simulink model "main_model"  (R2021b)
settings: Solver=ode4  StartTime=0.0  StopTime=7.0  FixedStep=rmpcProps.time_step  RelTol=1e-3
undefined symbols (not defined in the file): driverProps, refTraj, rmpcProps, vehProps
settings Model: Creator=vpurohi  LastModifiedBy=vpurohi

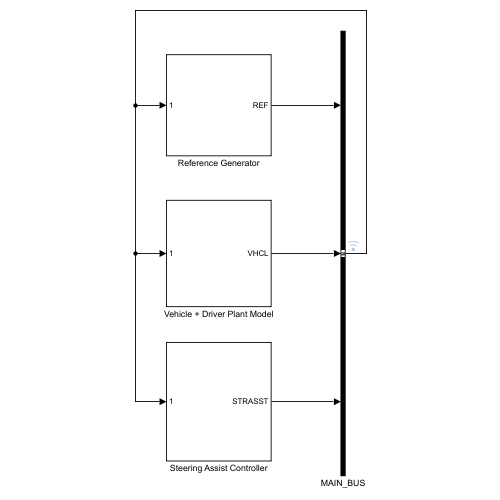
[thumbnail: Simulink's stored preview of the top-level diagram]
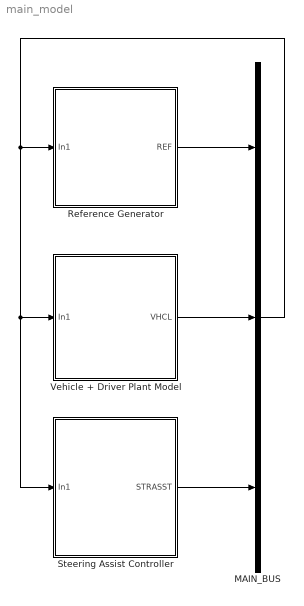
== system main_model ==
  MAIN_BUS : BusCreator  Inputs=3
  Reference Generator : Subsystem
  Steering Assist Controller : Subsystem
  Vehicle + Driver Plant Model : Subsystem
  wires:
  Reference Generator/1(REF) -> MAIN_BUS/1
  Vehicle + Driver Plant Model/1(VHCL) -> MAIN_BUS/2
  MAIN_BUS/1 -> Steering Assist Controller/1(In1), Vehicle + Driver Plant Model/1(In1), Reference Generator/1(In1)
  Steering Assist Controller/1(STRASST) -> MAIN_BUS/3

== system main_model/Reference Generator ==
  In1 : Inport
  1-D Lookup Table : Lookup_n-D  NumberOfTableDimensions=1  BreakpointsForDimension1=refTraj.X  Table=refTraj.psi_ref  InterpMethod=Akima spline  InternalRulePriority=Speed  RndMeth=Simplest  InputSameDT=on
  Add1 : Sum
  Bus Selector : BusSelector  OutputSignals=VHCL.X
  Constant : Constant  Value=driverProps.La
  reference : BusCreator  Inputs=1
  REF : Outport
  wires:
  Bus Selector/1 -> Add1/1  "<X>"
  Add1/1 -> 1-D Lookup Table/1
  Constant/1 -> Add1/2
  In1/1 -> Bus Selector/1
  1-D Lookup Table/1 -> reference/1  "psi_ref"
  reference/1 -> REF/1  "REF"

== system main_model/Steering Assist Controller ==
  In1 : Inport
  Bus Creator1 : BusCreator  Inputs=2
  Bus Selector : BusSelector  OutputSignals=VHCL.beta,VHCL.r,VHCL.delta_dr,VHCL.psi,VHCL.delta_y,VHCL.X,VHCL.Y
  Controller : MATLAB Function  TreatAsAtomicUnit=on  mask{vehProps=vehProps, driverProps=driverProps, controlProps=rmpcProps, refTraj=refTraj}
      mask prompts: vehProps "Vehicle Properties"; driverProps "Driver Properties"; controlProps "Control Properties"; refTraj "Reference Trajectory"
  Memory1 : Memory
  Mux : Mux  Inputs=2
  Mux1 : Mux  Inputs=7
  STRASST : Outport
  wires:
  Bus Creator1/1 -> STRASST/1  "STRASST"
  In1/1 -> Bus Selector/1
  Mux/1 -> Memory1/1
  Controller/1(u_ctrl) -> Mux/1, Bus Creator1/1
  Memory1/1 -> Controller/2(U0)
  Controller/2(sv) -> Bus Creator1/2, Mux/2
  Bus Selector/1 -> Mux1/1  "<beta>"
  Bus Selector/2 -> Mux1/2  "<r>"
  Bus Selector/3 -> Mux1/3  "<delta_dr>"
  Bus Selector/4 -> Mux1/4  "<psi>"
  Bus Selector/5 -> Mux1/5  "<delta_y>"
  Bus Selector/6 -> Mux1/6  "<X>"
  Bus Selector/7 -> Mux1/7  "<Y>"
  Mux1/1 -> Controller/1(x0)  "x0"

== system main_model/Vehicle + Driver Plant Model ==
  In1 : Inport
  Bicycle Model with Front Steering : Subsystem
  Bus Selector : BusSelector  OutputSignals=VHCL.delta_dr,STRASST.u_ctrl,VHCL.r,REF.psi_ref,VHCL.beta,VHCL.psi
  Driver Model : Subsystem
  To Workspace : ToWorkspace  VariableName=X  SampleTime=-1
  To Workspace1 : ToWorkspace  VariableName=Y  SampleTime=-1
  To Workspace2 : ToWorkspace  VariableName=footprint  SampleTime=-1
  Vehicle Trajectory & Footprint : Subsystem
  vehicle : BusCreator  Inputs=11
  vehicle1 : BusCreator  Inputs=8
  VHCL : Outport
  wires:
  Bicycle Model with Front Steering/2(r) -> vehicle/2  "r"
  Vehicle Trajectory & Footprint/1(X) -> To Workspace/1, vehicle/9  "X"
  Bicycle Model with Front Steering/1(beta) -> vehicle/1  "beta"
  Vehicle Trajectory & Footprint/2(Y) -> To Workspace1/1, vehicle/10  "Y"
  Bicycle Model with Front Steering/3(alpha_fr) -> vehicle/3  "alpha_fr"
  Bicycle Model with Front Steering/4(alpha_rr) -> vehicle/4  "alpha_rr"
  vehicle/1 -> VHCL/1  "VHCL"
  In1/1 -> Bus Selector/1
  vehicle1/1 -> To Workspace2/1, vehicle/11  "footprint"
  Bus Selector/1 -> Bicycle Model with Front Steering/1(delta_dr)  "<delta_dr>"
  Bus Selector/3 -> Driver Model/1(r)  "<r>"
  Bus Selector/5 -> Driver Model/3(beta), Vehicle Trajectory & Footprint/1(beta)  "<beta>"
  Bus Selector/6 -> Vehicle Trajectory & Footprint/2(psi)  "<psi>"
  Vehicle Trajectory & Footprint/3(x_fr) -> vehicle1/1
  Vehicle Trajectory & Footprint/4(x_fl) -> vehicle1/2
  Vehicle Trajectory & Footprint/5(x_rr) -> vehicle1/3
  Vehicle Trajectory & Footprint/6(x_rl) -> vehicle1/4
  Vehicle Trajectory & Footprint/7(y_fr) -> vehicle1/5
  Vehicle Trajectory & Footprint/8(y_fl) -> vehicle1/6
  Vehicle Trajectory & Footprint/9(y_rr) -> vehicle1/7
  Vehicle Trajectory & Footprint/10(y_rl) -> vehicle1/8
  Driver Model/1(psi) -> vehicle/6  "psi"
  Driver Model/2(delta_dr) -> vehicle/7  "delta_dr"
  Bus Selector/4 -> Driver Model/2(psi_ref)  "<psi_ref>"
  Bus Selector/2 -> Bicycle Model with Front Steering/2(u_ctrl)  "<u_ctrl>"
  Driver Model/3(delta_y) -> vehicle/8  "delta_y"
  Bicycle Model with Front Steering/5(delta_total) -> vehicle/5  "delta_total"

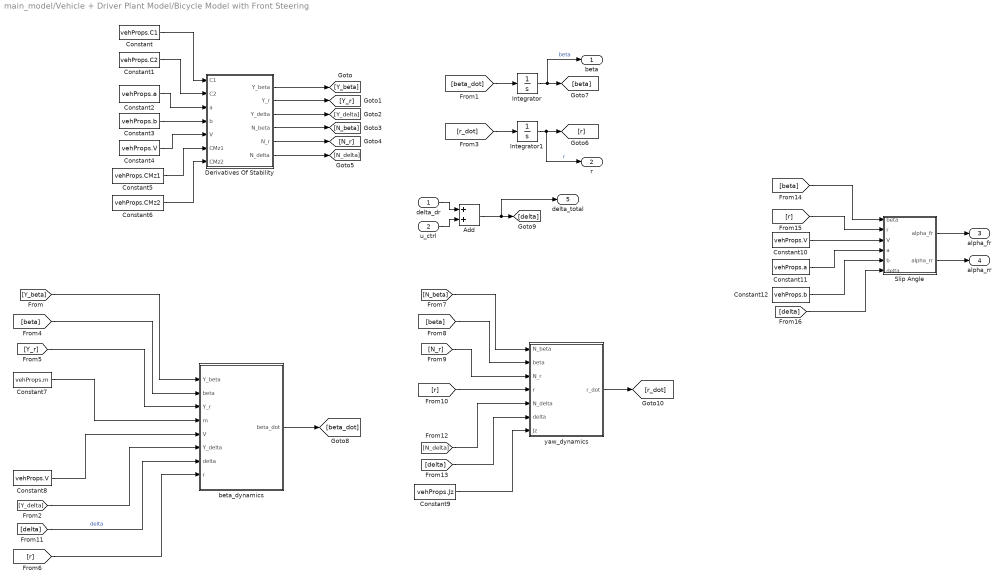
== system main_model/Vehicle + Driver Plant Model/Bicycle Model with Front Steering ==
  delta_dr : Inport
  u_ctrl : Inport  Port=2
  Add : Sum
  Constant : Constant  Value=vehProps.C1
  Constant1 : Constant  Value=vehProps.C2
  Constant10 : Constant  Value=vehProps.V
  Constant11 : Constant  Value=vehProps.a
  Constant12 : Constant  Value=vehProps.b
  Constant2 : Constant  Value=vehProps.a
  Constant3 : Constant  Value=vehProps.b
  Constant4 : Constant  Value=vehProps.V
  Constant5 : Constant  Value=vehProps.CMz1
  Constant6 : Constant  Value=vehProps.CMz2
  Constant7 : Constant  Value=vehProps.m
  Constant8 : Constant  Value=vehProps.V
  Constant9 : Constant  Value=vehProps.Jz
  Derivatives Of Stability : Subsystem
  Integrator : Integrator
  Integrator1 : Integrator
  Slip Angle : Subsystem
  beta_dynamics : Subsystem
  yaw_dynamics : Subsystem
  beta : Outport
  r : Outport  Port=2
  alpha_fr : Outport  Port=3
  alpha_rr : Outport  Port=4
  delta_total : Outport  Port=5
  wires:
  [r] -> beta_dynamics/8(r)
  Derivatives Of Stability/5(N_r) -> [N_r]
  Derivatives Of Stability/2(Y_r) -> [Y_r]
  [Y_beta] -> beta_dynamics/1(Y_beta)
  Constant5/1 -> Derivatives Of Stability/6(CMz1)
  yaw_dynamics/1(r_dot) -> [r_dot]
  Constant9/1 -> yaw_dynamics/7(Jz)
  [r_dot] -> Integrator1/1
  Derivatives Of Stability/3(Y_delta) -> [Y_delta]
  Integrator1/1 -> r/1, [r]  "r"
  [beta] -> yaw_dynamics/2(beta)
  Integrator/1 -> beta/1, [beta]  "beta"
  [delta] -> beta_dynamics/7(delta)  "delta"
  Constant4/1 -> Derivatives Of Stability/5(V)
  Derivatives Of Stability/4(N_beta) -> [N_beta]
  [beta] -> beta_dynamics/2(beta)
  [Y_r] -> beta_dynamics/3(Y_r)
  Constant8/1 -> beta_dynamics/5(V)
  [N_delta] -> yaw_dynamics/5(N_delta)
  Derivatives Of Stability/1(Y_beta) -> [Y_beta]
  Constant7/1 -> beta_dynamics/4(m)
  [Y_delta] -> beta_dynamics/6(Y_delta)
  beta_dynamics/1(beta_dot) -> [beta_dot]
  Constant3/1 -> Derivatives Of Stability/4(b)
  Constant1/1 -> Derivatives Of Stability/2(C2)
  [beta_dot] -> Integrator/1
  [N_beta] -> yaw_dynamics/1(N_beta)
  Derivatives Of Stability/6(N_delta) -> [N_delta]
  Constant6/1 -> Derivatives Of Stability/7(CMz2)
  Constant/1 -> Derivatives Of Stability/1(C1)
  Constant2/1 -> Derivatives Of Stability/3(a)
  [N_r] -> yaw_dynamics/3(N_r)
  [r] -> yaw_dynamics/4(r)
  [delta] -> yaw_dynamics/6(delta)
  [beta] -> Slip Angle/1(beta)
  [r] -> Slip Angle/2(r)
  Constant10/1 -> Slip Angle/3(V)
  Constant11/1 -> Slip Angle/4(a)
  Slip Angle/1(alpha_fr) -> alpha_fr/1
  [delta] -> Slip Angle/6(delta)
  Constant12/1 -> Slip Angle/5(b)
  Slip Angle/2(alpha_rr) -> alpha_rr/1
  delta_dr/1 -> Add/1
  u_ctrl/1 -> Add/2
  Add/1 -> delta_total/1, [delta]

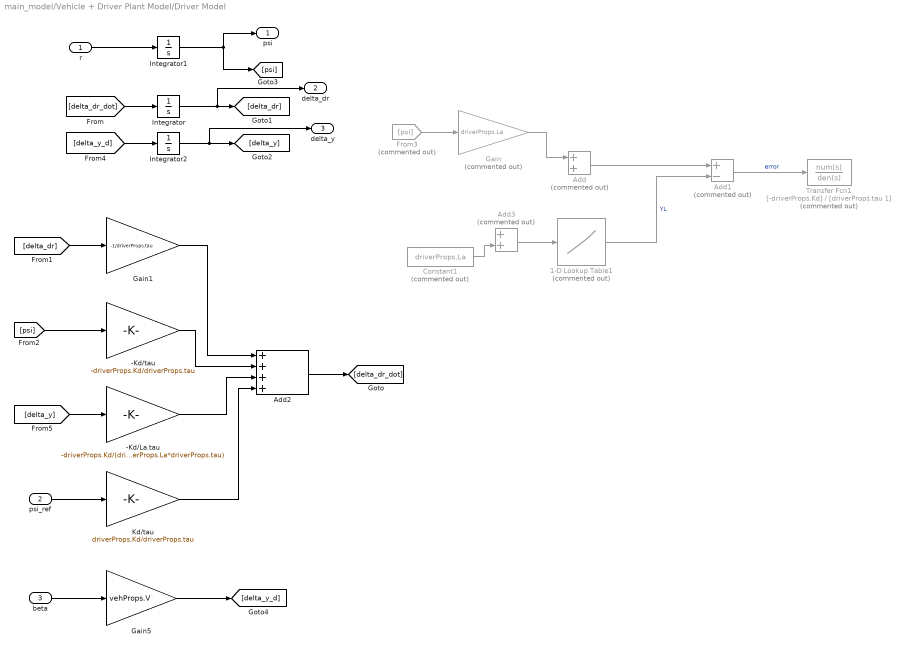
== system main_model/Vehicle + Driver Plant Model/Driver Model ==
  r : Inport
  psi_ref : Inport  Port=2
  beta : Inport  Port=3
  -Kd/La.tau : Gain  Gain=-driverProps.Kd/(driverProps.La*driverProps.tau)
  -Kd/tau : Gain  Gain=-driverProps.Kd/driverProps.tau
  1-D Lookup Table1 : Lookup_n-D  Commented=on  NumberOfTableDimensions=1  BreakpointsForDimension1=refTraj.X  Table=refTraj.Y  InterpMethod=Akima spline  ExtrapMethod=Clip  UseLastTableValue=on  InternalRulePriority=Speed  RndMeth=Simplest  InputSameDT=on
  Add : Sum  Commented=on
  Add1 : Sum  Commented=on  Inputs=+-
  Add2 : Sum  Inputs=++++
  Add3 : Sum  Commented=on
  Constant1 : Constant  Commented=on  Value=driverProps.La
  From3 : From  Commented=on  GotoTag=psi
  Gain : Gain  Commented=on  Gain=driverProps.La
  Gain1 : Gain  Gain=-1/driverProps.tau
  Gain5 : Gain  Gain=vehProps.V
  Integrator : Integrator
  Integrator1 : Integrator
  Integrator2 : Integrator
  Kd/tau : Gain  Gain=driverProps.Kd/driverProps.tau
  Transfer Fcn1 : TransferFcn  Commented=on  Numerator=[-driverProps.Kd]  Denominator=[driverProps.tau 1]
  psi : Outport
  delta_dr : Outport  Port=2
  delta_y : Outport  Port=3
  wires:
  Integrator1/1 -> psi/1, [psi]
  r/1 -> Integrator1/1
  Add1/1 -> Transfer Fcn1/1  "error"
  1-D Lookup Table1/1 -> Add1/2  "YL"
  Constant1/1 -> Add3/2
  Add/1 -> Add1/1
  Gain/1 -> Add/1
  Add3/1 -> 1-D Lookup Table1/1
  From3/1 -> Gain/1
  [delta_dr_dot] -> Integrator/1
  Integrator/1 -> delta_dr/1, [delta_dr]
  [delta_dr] -> Gain1/1
  [psi] -> -Kd/tau/1
  [delta_y_d] -> Integrator2/1
  Integrator2/1 -> delta_y/1, [delta_y]
  [delta_y] -> -Kd/La.tau/1
  psi_ref/1 -> Kd/tau/1
  Gain1/1 -> Add2/1
  -Kd/tau/1 -> Add2/2
  -Kd/La.tau/1 -> Add2/3
  Kd/tau/1 -> Add2/4
  Add2/1 -> [delta_dr_dot]
  beta/1 -> Gain5/1
  Gain5/1 -> [delta_y_d]

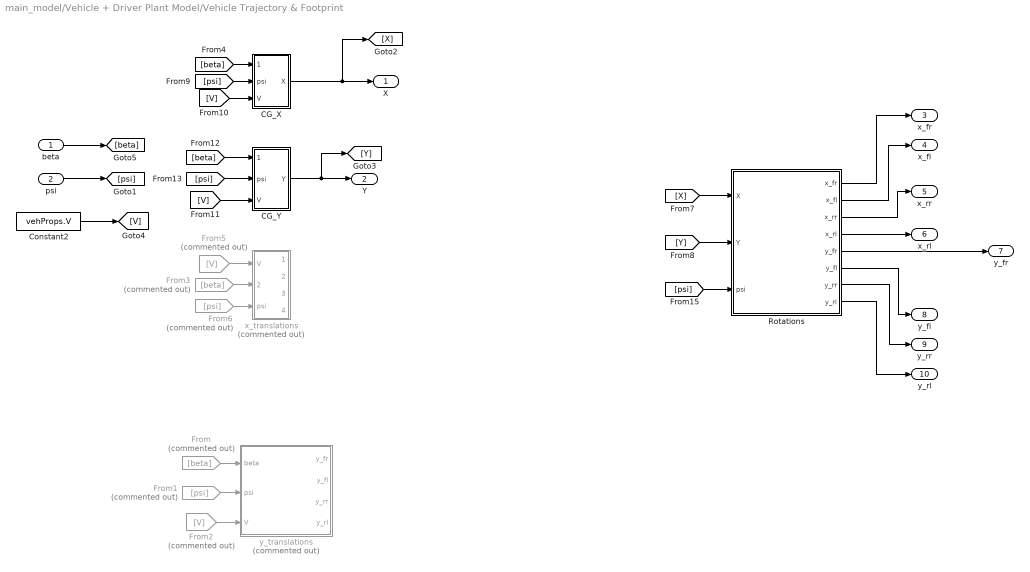
== system main_model/Vehicle + Driver Plant Model/Vehicle Trajectory & Footprint ==
  beta : Inport
  psi : Inport  Port=2
  CG_X : Subsystem
  CG_Y : Subsystem
  Constant2 : Constant  Value=vehProps.V
  From : From  Commented=on  GotoTag=beta
  From1 : From  Commented=on  GotoTag=psi
  From2 : From  Commented=on  GotoTag=V
  From3 : From  Commented=on  GotoTag=beta
  From5 : From  Commented=on  GotoTag=V
  From6 : From  Commented=on  GotoTag=psi
  Rotations : Subsystem
  x_translations : Subsystem  Commented=on
  y_translations : Subsystem  Commented=on
  X : Outport
  Y : Outport  Port=2
  x_fr : Outport  Port=3
  x_fl : Outport  Port=4
  x_rr : Outport  Port=5
  x_rl : Outport  Port=6
  y_fr : Outport  Port=7
  y_fl : Outport  Port=8
  y_rr : Outport  Port=9
  y_rl : Outport  Port=10
  wires:
  Constant2/1 -> [V]
  CG_X/1(X) -> [X], X/1
  From5/1 -> x_translations/1(V)
  From/1 -> y_translations/1(beta)
  From1/1 -> y_translations/2(psi)
  From2/1 -> y_translations/3(V)
  From3/1 -> x_translations/2(beta)
  From6/1 -> x_translations/3(psi)
  Rotations/1(x_fr) -> x_fr/1
  Rotations/2(x_fl) -> x_fl/1
  Rotations/3(x_rr) -> x_rr/1
  Rotations/4(x_rl) -> x_rl/1
  Rotations/5(y_fr) -> y_fr/1
  Rotations/6(y_fl) -> y_fl/1
  Rotations/7(y_rr) -> y_rr/1
  Rotations/8(y_rl) -> y_rl/1
  [psi] -> Rotations/3(psi)
  [X] -> Rotations/1(X)
  [Y] -> Rotations/2(Y)
  psi/1 -> [psi]
  beta/1 -> [beta]
  [beta] -> CG_X/1(beta)
  [psi] -> CG_X/2(psi)
  [V] -> CG_X/3(V)
  [beta] -> CG_Y/1(beta)
  [psi] -> CG_Y/2(psi)
  [V] -> CG_Y/3(V)
  CG_Y/1(Y) -> [Y], Y/1

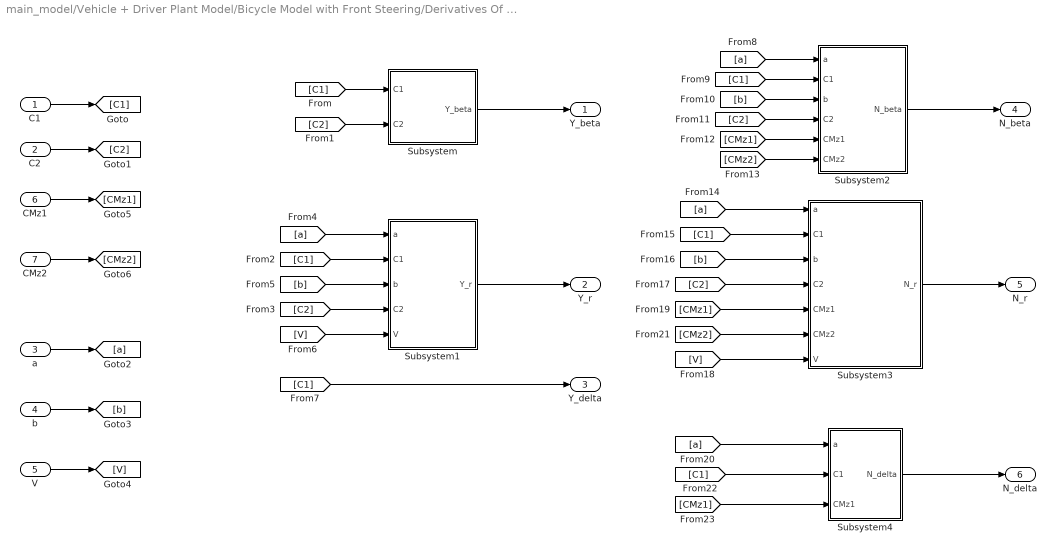
== system main_model/Vehicle + Driver Plant Model/Bicycle Model with Front Steering/Derivatives Of Stability ==
  C1 : Inport
  C2 : Inport  Port=2
  a : Inport  Port=3
  b : Inport  Port=4
  V : Inport  Port=5
  CMz1 : Inport  Port=6
  CMz2 : Inport  Port=7
  Subsystem : Subsystem
  Subsystem1 : Subsystem
  Subsystem2 : Subsystem
  Subsystem3 : Subsystem
  Subsystem4 : Subsystem
  Y_beta : Outport
  Y_r : Outport  Port=2
  Y_delta : Outport  Port=3
  N_beta : Outport  Port=4
  N_r : Outport  Port=5
  N_delta : Outport  Port=6
  wires:
  Subsystem2/1(N_beta) -> N_beta/1
  Subsystem/1(Y_beta) -> Y_beta/1
  [CMz1] -> Subsystem4/3(CMz1)
  C2/1 -> [C2]
  [C2] -> Subsystem1/4(C2)
  Subsystem3/1(N_r) -> N_r/1
  b/1 -> [b]
  Subsystem4/1(N_delta) -> N_delta/1
  [a] -> Subsystem3/1(a)
  C1/1 -> [C1]
  [a] -> Subsystem2/1(a)
  a/1 -> [a]
  [C2] -> Subsystem2/4(C2)
  [b] -> Subsystem1/3(b)
  CMz1/1 -> [CMz1]
  Subsystem1/1(Y_r) -> Y_r/1
  CMz2/1 -> [CMz2]
  [V] -> Subsystem1/5(V)
  [C2] -> Subsystem/2(C2)
  [C1] -> Y_delta/1
  V/1 -> [V]
  [C1] -> Subsystem2/2(C1)
  [V] -> Subsystem3/7(V)
  [C1] -> Subsystem/1(C1)
  [a] -> Subsystem1/1(a)
  [C2] -> Subsystem3/4(C2)
  [a] -> Subsystem4/1(a)
  [CMz2] -> Subsystem3/6(CMz2)
  [CMz1] -> Subsystem3/5(CMz1)
  [CMz2] -> Subsystem2/6(CMz2)
  [C1] -> Subsystem3/2(C1)
  [C1] -> Subsystem1/2(C1)
  [b] -> Subsystem2/3(b)
  [CMz1] -> Subsystem2/5(CMz1)
  [b] -> Subsystem3/3(b)
  [C1] -> Subsystem4/2(C1)

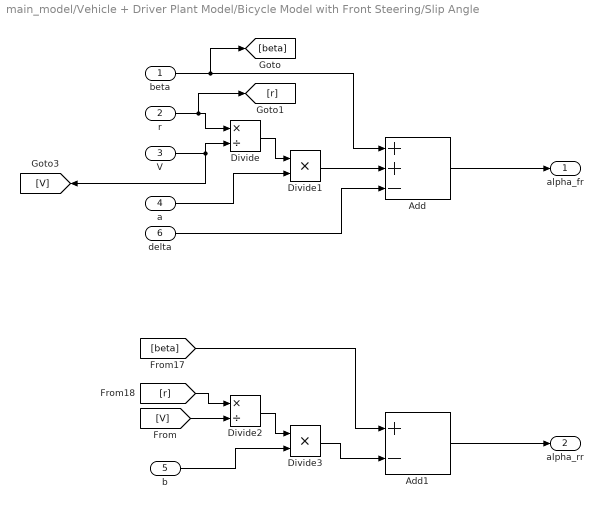
== system main_model/Vehicle + Driver Plant Model/Bicycle Model with Front Steering/Slip Angle ==
  beta : Inport
  r : Inport  Port=2
  V : Inport  Port=3
  a : Inport  Port=4
  b : Inport  Port=5
  delta : Inport  Port=6
  Add : Sum  Inputs=++-
  Add1 : Sum  Inputs=+-
  Divide : Product  Inputs=*/
  Divide1 : Product  Inputs=**
  Divide2 : Product  Inputs=*/
  Divide3 : Product  Inputs=**
  alpha_fr : Outport
  alpha_rr : Outport  Port=2
  wires:
  V/1 -> Divide/2, [V]
  r/1 -> [r], Divide/1
  Divide1/1 -> Add/2
  Divide/1 -> Divide1/1
  Add/1 -> alpha_fr/1
  a/1 -> Divide1/2
  beta/1 -> [beta], Add/1
  Divide3/1 -> Add1/2
  b/1 -> Divide3/2
  [beta] -> Add1/1
  [r] -> Divide2/1
  Divide2/1 -> Divide3/1
  delta/1 -> Add/3
  [V] -> Divide2/2
  Add1/1 -> alpha_rr/1

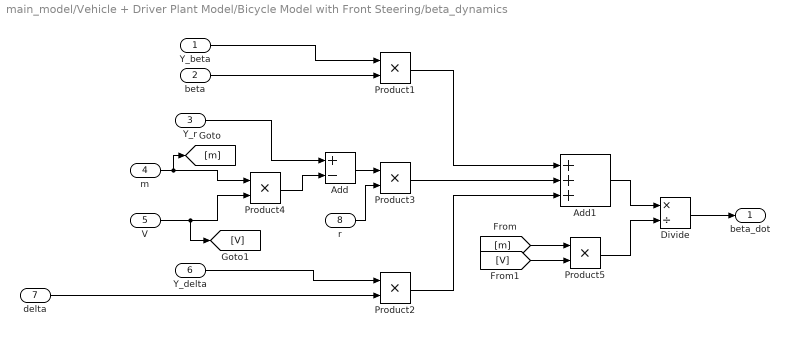
== system main_model/Vehicle + Driver Plant Model/Bicycle Model with Front Steering/beta_dynamics ==
  Y_beta : Inport
  beta : Inport  Port=2
  Y_r : Inport  Port=3
  m : Inport  Port=4
  V : Inport  Port=5
  Y_delta : Inport  Port=6
  delta : Inport  Port=7
  r : Inport  Port=8
  Add : Sum  Inputs=+-
  Add1 : Sum  Inputs=+++
  Divide : Product  Inputs=*/
  Product{1..5} (5 alike) : Product
  beta_dot : Outport
  wires:
  Product2/1 -> Add1/3
  Add1/1 -> Divide/1
  Product3/1 -> Add1/2
  Product4/1 -> Add/2
  delta/1 -> Product2/2
  Add/1 -> Product3/1
  Product1/1 -> Add1/1
  r/1 -> Product3/2
  m/1 -> [m], Product4/1
  Y_delta/1 -> Product2/1
  Product5/1 -> Divide/2
  Y_beta/1 -> Product1/1
  V/1 -> [V], Product4/2
  Divide/1 -> beta_dot/1
  beta/1 -> Product1/2
  Y_r/1 -> Add/1
  [m] -> Product5/1
  [V] -> Product5/2

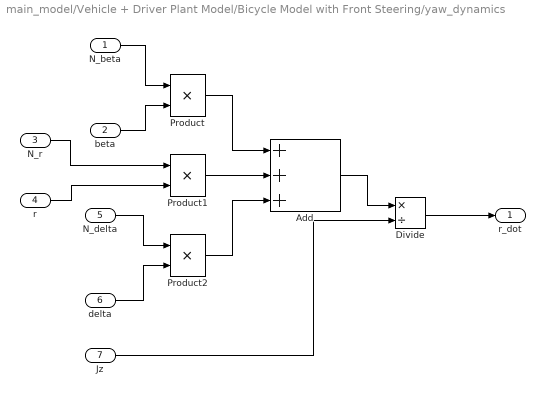
== system main_model/Vehicle + Driver Plant Model/Bicycle Model with Front Steering/yaw_dynamics ==
  N_beta : Inport
  beta : Inport  Port=2
  N_r : Inport  Port=3
  r : Inport  Port=4
  N_delta : Inport  Port=5
  delta : Inport  Port=6
  Jz : Inport  Port=7
  Add : Sum  Inputs=+++
  Divide : Product  Inputs=*/
  Product : Product
  Product1 : Product
  Product2 : Product
  r_dot : Outport
  wires:
  r/1 -> Product1/2
  Product2/1 -> Add/3
  delta/1 -> Product2/2
  Add/1 -> Divide/1
  beta/1 -> Product/2
  Divide/1 -> r_dot/1
  N_r/1 -> Product1/1
  Product1/1 -> Add/2
  Product/1 -> Add/1
  N_delta/1 -> Product2/1
  N_beta/1 -> Product/1
  Jz/1 -> Divide/2

== system main_model/Vehicle + Driver Plant Model/Vehicle Trajectory & Footprint/CG_X ==
  beta : Inport
  psi : Inport  Port=2
  V : Inport  Port=3
  Add : Sum
  Cos : Trigonometry  Operator=cos
  Integrator : Integrator
  Product : Product
  X : Outport
  wires:
  Integrator/1 -> X/1
  beta/1 -> Add/1
  psi/1 -> Add/2
  Add/1 -> Cos/1
  Cos/1 -> Product/1
  V/1 -> Product/2
  Product/1 -> Integrator/1

== system main_model/Vehicle + Driver Plant Model/Vehicle Trajectory & Footprint/CG_Y ==
  beta : Inport
  psi : Inport  Port=2
  V : Inport  Port=3
  Add : Sum
  Cos : Trigonometry
  Integrator : Integrator
  Product : Product
  Y : Outport
  wires:
  psi/1 -> Add/2
  Cos/1 -> Product/1
  beta/1 -> Add/1
  Integrator/1 -> Y/1
  Product/1 -> Integrator/1
  Add/1 -> Cos/1
  V/1 -> Product/2

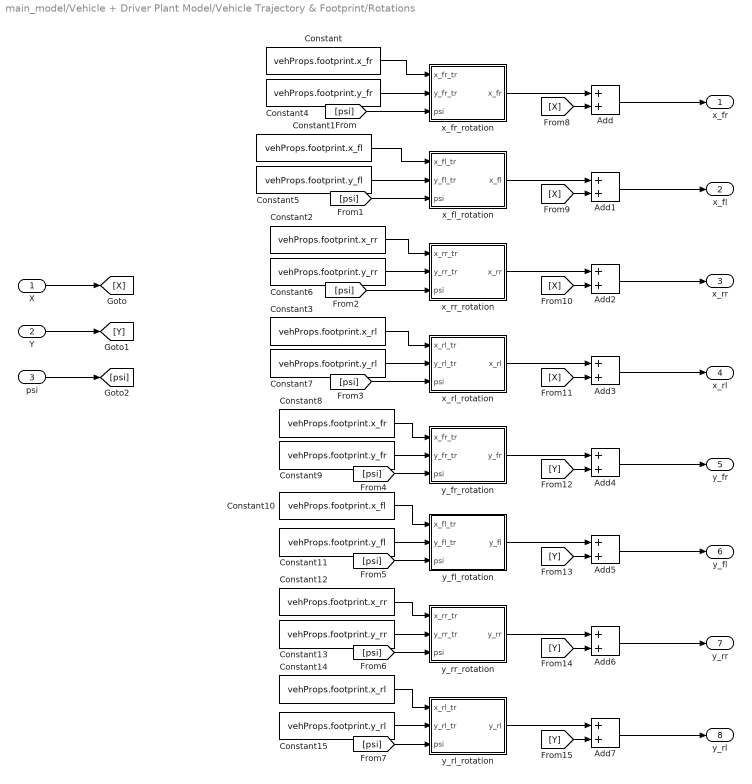
== system main_model/Vehicle + Driver Plant Model/Vehicle Trajectory & Footprint/Rotations ==
  X : Inport
  Y : Inport  Port=2
  psi : Inport  Port=3
  Add{,1..7} (8 alike) : Sum
  Constant : Constant  Value=vehProps.footprint.x_fr
  Constant1 : Constant  Value=vehProps.footprint.x_fl
  Constant10 : Constant  Value=vehProps.footprint.x_fl
  Constant11 : Constant  Value=vehProps.footprint.y_fl
  Constant12 : Constant  Value=vehProps.footprint.x_rr
  Constant13 : Constant  Value=vehProps.footprint.y_rr
  Constant14 : Constant  Value=vehProps.footprint.x_rl
  Constant15 : Constant  Value=vehProps.footprint.y_rl
  Constant2 : Constant  Value=vehProps.footprint.x_rr
  Constant3 : Constant  Value=vehProps.footprint.x_rl
  Constant4 : Constant  Value=vehProps.footprint.y_fr
  Constant5 : Constant  Value=vehProps.footprint.y_fl
  Constant6 : Constant  Value=vehProps.footprint.y_rr
  Constant7 : Constant  Value=vehProps.footprint.y_rl
  Constant8 : Constant  Value=vehProps.footprint.x_fr
  Constant9 : Constant  Value=vehProps.footprint.y_fr
  x_fl_rotation : Subsystem
  x_fr_rotation : Subsystem
  x_rl_rotation : Subsystem
  x_rr_rotation : Subsystem
  y_fl_rotation : Subsystem
  y_fr_rotation : Subsystem
  y_rl_rotation : Subsystem
  y_rr_rotation : Subsystem
  x_fr : Outport
  x_fl : Outport  Port=2
  x_rr : Outport  Port=3
  x_rl : Outport  Port=4
  y_fr : Outport  Port=5
  y_fl : Outport  Port=6
  y_rr : Outport  Port=7
  y_rl : Outport  Port=8
  wires:
  Constant/1 -> x_fr_rotation/1(x_fr_tr)
  Constant4/1 -> x_fr_rotation/2(y_fr_tr)
  [psi] -> x_fr_rotation/3(psi)
  Constant1/1 -> x_fl_rotation/1(x_fl_tr)
  Constant5/1 -> x_fl_rotation/2(y_fl_tr)
  [psi] -> x_fl_rotation/3(psi)
  Constant2/1 -> x_rr_rotation/1(x_rr_tr)
  Constant6/1 -> x_rr_rotation/2(y_rr_tr)
  [psi] -> x_rr_rotation/3(psi)
  Constant3/1 -> x_rl_rotation/1(x_rl_tr)
  Constant7/1 -> x_rl_rotation/2(y_rl_tr)
  [psi] -> x_rl_rotation/3(psi)
  Constant8/1 -> y_fr_rotation/1(x_fr_tr)
  Constant9/1 -> y_fr_rotation/2(y_fr_tr)
  [psi] -> y_fr_rotation/3(psi)
  Constant10/1 -> y_fl_rotation/1(x_fl_tr)
  Constant11/1 -> y_fl_rotation/2(y_fl_tr)
  [psi] -> y_fl_rotation/3(psi)
  Constant12/1 -> y_rr_rotation/1(x_rr_tr)
  Constant13/1 -> y_rr_rotation/2(y_rr_tr)
  [psi] -> y_rr_rotation/3(psi)
  Constant14/1 -> y_rl_rotation/1(x_rl_tr)
  Constant15/1 -> y_rl_rotation/2(y_rl_tr)
  [psi] -> y_rl_rotation/3(psi)
  X/1 -> [X]
  Y/1 -> [Y]
  Add/1 -> x_fr/1
  x_fr_rotation/1(x_fr) -> Add/1
  x_fl_rotation/1(x_fl) -> Add1/1
  Add1/1 -> x_fl/1
  x_rr_rotation/1(x_rr) -> Add2/1
  Add2/1 -> x_rr/1
  x_rl_rotation/1(x_rl) -> Add3/1
  Add3/1 -> x_rl/1
  y_fr_rotation/1(y_fr) -> Add4/1
  Add4/1 -> y_fr/1
  y_fl_rotation/1(y_fl) -> Add5/1
  Add5/1 -> y_fl/1
  y_rr_rotation/1(y_rr) -> Add6/1
  Add6/1 -> y_rr/1
  y_rl_rotation/1(y_rl) -> Add7/1
  Add7/1 -> y_rl/1
  [X] -> Add/2
  [X] -> Add1/2
  [X] -> Add2/2
  [X] -> Add3/2
  [Y] -> Add4/2
  [Y] -> Add5/2
  [Y] -> Add6/2
  [Y] -> Add7/2
  psi/1 -> [psi]

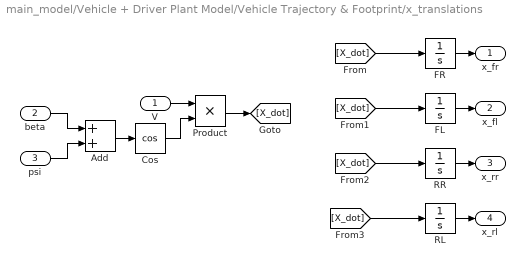
== system main_model/Vehicle + Driver Plant Model/Vehicle Trajectory & Footprint/x_translations ==
  V : Inport
  beta : Inport  Port=2
  psi : Inport  Port=3
  Add : Sum
  Cos : Trigonometry  Operator=cos
  FL : Integrator  InitialCondition=vehProps.footprint.x_fl
  FR : Integrator  InitialCondition=vehProps.footprint.x_fr
  Product : Product
  RL : Integrator  InitialCondition=vehProps.footprint.x_rl
  RR : Integrator  InitialCondition=vehProps.footprint.x_rr
  x_fr : Outport
  x_fl : Outport  Port=2
  x_rr : Outport  Port=3
  x_rl : Outport  Port=4
  wires:
  RL/1 -> x_rl/1
  RR/1 -> x_rr/1
  FL/1 -> x_fl/1
  FR/1 -> x_fr/1
  beta/1 -> Add/1
  psi/1 -> Add/2
  Add/1 -> Cos/1
  Cos/1 -> Product/2
  V/1 -> Product/1
  Product/1 -> [X_dot]
  [X_dot] -> FR/1
  [X_dot] -> FL/1
  [X_dot] -> RR/1
  [X_dot] -> RL/1

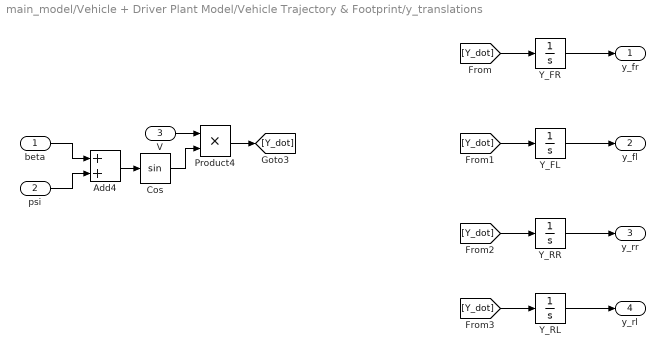
== system main_model/Vehicle + Driver Plant Model/Vehicle Trajectory & Footprint/y_translations ==
  beta : Inport
  psi : Inport  Port=2
  V : Inport  Port=3
  Add4 : Sum
  Cos : Trigonometry
  Product4 : Product
  Y_FL : Integrator  InitialCondition=vehProps.footprint.y_fl
  Y_FR : Integrator  InitialCondition=vehProps.footprint.y_fr
  Y_RL : Integrator  InitialCondition=vehProps.footprint.y_rl
  Y_RR : Integrator  InitialCondition=vehProps.footprint.y_rr
  y_fr : Outport
  y_fl : Outport  Port=2
  y_rr : Outport  Port=3
  y_rl : Outport  Port=4
  wires:
  Y_RL/1 -> y_rl/1
  Y_FL/1 -> y_fl/1
  Y_RR/1 -> y_rr/1
  Y_FR/1 -> y_fr/1
  beta/1 -> Add4/1
  Cos/1 -> Product4/2
  Add4/1 -> Cos/1
  V/1 -> Product4/1
  Product4/1 -> [Y_dot]
  psi/1 -> Add4/2
  [Y_dot] -> Y_FR/1
  [Y_dot] -> Y_FL/1
  [Y_dot] -> Y_RR/1
  [Y_dot] -> Y_RL/1

== system main_model/Vehicle + Driver Plant Model/Bicycle Model with Front Steering/Derivatives Of Stability/Subsystem ==
  C1 : Inport
  C2 : Inport  Port=2
  Add : Sum
  Gain : Gain  Gain=-1
  Y_beta : Outport
  wires:
  Add/1 -> Gain/1
  C1/1 -> Add/1
  Gain/1 -> Y_beta/1
  C2/1 -> Add/2

== system main_model/Vehicle + Driver Plant Model/Bicycle Model with Front Steering/Derivatives Of Stability/Subsystem1 ==
  a : Inport
  C1 : Inport  Port=2
  b : Inport  Port=3
  C2 : Inport  Port=4
  V : Inport  Port=5
  Add1 : Sum  Inputs=+-
  Divide : Product  Inputs=*/
  Gain1 : Gain  Gain=-1
  Product : Product
  Product1 : Product
  Y_r : Outport
  wires:
  Gain1/1 -> Divide/2
  Product/1 -> Add1/1
  Add1/1 -> Divide/1
  C1/1 -> Product/2
  Product1/1 -> Add1/2
  Divide/1 -> Y_r/1
  b/1 -> Product1/1
  C2/1 -> Product1/2
  V/1 -> Gain1/1
  a/1 -> Product/1

== system main_model/Vehicle + Driver Plant Model/Bicycle Model with Front Steering/Derivatives Of Stability/Subsystem2 ==
  a : Inport
  C1 : Inport  Port=2
  b : Inport  Port=3
  C2 : Inport  Port=4
  CMz1 : Inport  Port=5
  CMz2 : Inport  Port=6
  Add2 : Sum  Inputs=++++
  Gain2 : Gain  Gain=-1
  Product2 : Product
  Product3 : Product
  N_beta : Outport
  wires:
  C1/1 -> Product2/2
  Add2/1 -> N_beta/1
  Product3/1 -> Add2/2
  CMz1/1 -> Add2/3
  a/1 -> Gain2/1
  Product2/1 -> Add2/1
  CMz2/1 -> Add2/4
  Gain2/1 -> Product2/1
  b/1 -> Product3/1
  C2/1 -> Product3/2

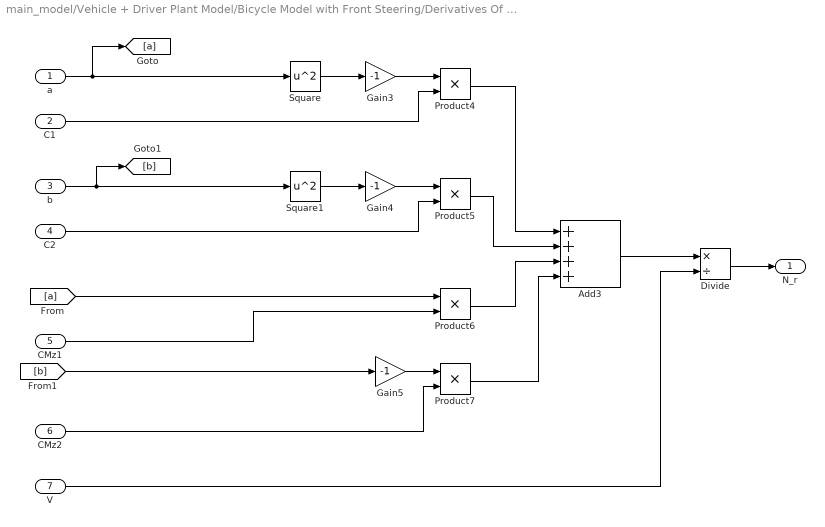
== system main_model/Vehicle + Driver Plant Model/Bicycle Model with Front Steering/Derivatives Of Stability/Subsystem3 ==
  a : Inport
  C1 : Inport  Port=2
  b : Inport  Port=3
  C2 : Inport  Port=4
  CMz1 : Inport  Port=5
  CMz2 : Inport  Port=6
  V : Inport  Port=7
  Add3 : Sum  Inputs=++++
  Divide : Product  Inputs=*/
  Gain3 : Gain  Gain=-1
  Gain4 : Gain  Gain=-1
  Gain5 : Gain  Gain=-1
  Product{4..7} (4 alike) : Product
  Square : Math  Operator=square  SaturateOnIntegerOverflow=on
  Square1 : Math  Operator=square  SaturateOnIntegerOverflow=on
  N_r : Outport
  wires:
  a/1 -> [a], Square/1
  Gain5/1 -> Product7/1
  Gain3/1 -> Product4/1
  Gain4/1 -> Product5/1
  Square1/1 -> Gain4/1
  Product5/1 -> Add3/2
  Product6/1 -> Add3/3
  [b] -> Gain5/1
  Product4/1 -> Add3/1
  Square/1 -> Gain3/1
  Product7/1 -> Add3/4
  CMz1/1 -> Product6/2
  CMz2/1 -> Product7/2
  Add3/1 -> Divide/1
  C1/1 -> Product4/2
  b/1 -> [b], Square1/1
  C2/1 -> Product5/2
  [a] -> Product6/1
  V/1 -> Divide/2
  Divide/1 -> N_r/1

== system main_model/Vehicle + Driver Plant Model/Bicycle Model with Front Steering/Derivatives Of Stability/Subsystem4 ==
  a : Inport
  C1 : Inport  Port=2
  CMz1 : Inport  Port=3
  Add : Sum  Inputs=+-
  Product : Product
  N_delta : Outport
  wires:
  a/1 -> Product/1
  Product/1 -> Add/1
  CMz1/1 -> Add/2
  C1/1 -> Product/2
  Add/1 -> N_delta/1

== system main_model/Vehicle + Driver Plant Model/Vehicle Trajectory & Footprint/Rotations/x_fl_rotation ==
  x_fl_tr : Inport
  y_fl_tr : Inport  Port=2
  psi : Inport  Port=3
  Add : Sum  Inputs=+-
  Cos : Trigonometry  Operator=cos
  Cos1 : Trigonometry
  Product : Product
  Product1 : Product
  x_fl : Outport
  wires:
  Cos1/1 -> [sin_psi]
  [sin_psi] -> Product1/1
  [cos_psi] -> Product/1
  Product/1 -> Add/1
  Cos/1 -> [cos_psi]
  Product1/1 -> Add/2
  psi/1 -> Cos1/1, Cos/1
  x_fl_tr/1 -> Product/2
  y_fl_tr/1 -> Product1/2
  Add/1 -> x_fl/1

== system main_model/Vehicle + Driver Plant Model/Vehicle Trajectory & Footprint/Rotations/x_fr_rotation ==
  x_fr_tr : Inport
  y_fr_tr : Inport  Port=2
  psi : Inport  Port=3
  Add : Sum  Inputs=+-
  Cos : Trigonometry  Operator=cos
  Cos1 : Trigonometry
  Product : Product
  Product1 : Product
  x_fr : Outport
  wires:
  Cos1/1 -> [sin_psi]
  [sin_psi] -> Product1/1
  [cos_psi] -> Product/1
  Product/1 -> Add/1
  Cos/1 -> [cos_psi]
  Product1/1 -> Add/2
  psi/1 -> Cos1/1, Cos/1
  x_fr_tr/1 -> Product/2
  y_fr_tr/1 -> Product1/2
  Add/1 -> x_fr/1

== system main_model/Vehicle + Driver Plant Model/Vehicle Trajectory & Footprint/Rotations/x_rl_rotation ==
  x_rl_tr : Inport
  y_rl_tr : Inport  Port=2
  psi : Inport  Port=3
  Add : Sum  Inputs=+-
  Cos : Trigonometry  Operator=cos
  Cos1 : Trigonometry
  Product : Product
  Product1 : Product
  x_rl : Outport
  wires:
  Cos1/1 -> [sin_psi]
  [sin_psi] -> Product1/1
  [cos_psi] -> Product/1
  Product/1 -> Add/1
  Cos/1 -> [cos_psi]
  Product1/1 -> Add/2
  psi/1 -> Cos1/1, Cos/1
  x_rl_tr/1 -> Product/2
  y_rl_tr/1 -> Product1/2
  Add/1 -> x_rl/1

== system main_model/Vehicle + Driver Plant Model/Vehicle Trajectory & Footprint/Rotations/x_rr_rotation ==
  x_rr_tr : Inport
  y_rr_tr : Inport  Port=2
  psi : Inport  Port=3
  Add : Sum  Inputs=+-
  Cos : Trigonometry  Operator=cos
  Cos1 : Trigonometry
  Product : Product
  Product1 : Product
  x_rr : Outport
  wires:
  Cos1/1 -> [sin_psi]
  [sin_psi] -> Product1/1
  [cos_psi] -> Product/1
  Product/1 -> Add/1
  Cos/1 -> [cos_psi]
  Product1/1 -> Add/2
  psi/1 -> Cos1/1, Cos/1
  x_rr_tr/1 -> Product/2
  y_rr_tr/1 -> Product1/2
  Add/1 -> x_rr/1

== system main_model/Vehicle + Driver Plant Model/Vehicle Trajectory & Footprint/Rotations/y_fl_rotation ==
  x_fl_tr : Inport
  y_fl_tr : Inport  Port=2
  psi : Inport  Port=3
  Add : Sum
  Cos : Trigonometry  Operator=cos
  Cos1 : Trigonometry
  Product : Product
  Product1 : Product
  y_fl : Outport
  wires:
  Cos1/1 -> [sin_psi]
  Product/1 -> Add/1
  Cos/1 -> [cos_psi]
  Product1/1 -> Add/2
  psi/1 -> Cos1/1, Cos/1
  x_fl_tr/1 -> Product/2
  y_fl_tr/1 -> Product1/2
  Add/1 -> y_fl/1
  [cos_psi] -> Product1/1
  [sin_psi] -> Product/1

== system main_model/Vehicle + Driver Plant Model/Vehicle Trajectory & Footprint/Rotations/y_fr_rotation ==
  x_fr_tr : Inport
  y_fr_tr : Inport  Port=2
  psi : Inport  Port=3
  Add : Sum
  Cos : Trigonometry  Operator=cos
  Cos1 : Trigonometry
  Product : Product
  Product1 : Product
  y_fr : Outport
  wires:
  Cos1/1 -> [sin_psi]
  Product/1 -> Add/1
  Cos/1 -> [cos_psi]
  Product1/1 -> Add/2
  psi/1 -> Cos1/1, Cos/1
  x_fr_tr/1 -> Product/2
  y_fr_tr/1 -> Product1/2
  Add/1 -> y_fr/1
  [sin_psi] -> Product/1
  [cos_psi] -> Product1/1

== system main_model/Vehicle + Driver Plant Model/Vehicle Trajectory & Footprint/Rotations/y_rl_rotation ==
  x_rl_tr : Inport
  y_rl_tr : Inport  Port=2
  psi : Inport  Port=3
  Add : Sum
  Cos : Trigonometry  Operator=cos
  Cos1 : Trigonometry
  Product : Product
  Product1 : Product
  y_rl : Outport
  wires:
  Cos1/1 -> [sin_psi]
  Product/1 -> Add/1
  Cos/1 -> [cos_psi]
  Product1/1 -> Add/2
  psi/1 -> Cos1/1, Cos/1
  x_rl_tr/1 -> Product/2
  y_rl_tr/1 -> Product1/2
  Add/1 -> y_rl/1
  [cos_psi] -> Product1/1
  [sin_psi] -> Product/1

== system main_model/Vehicle + Driver Plant Model/Vehicle Trajectory & Footprint/Rotations/y_rr_rotation ==
  x_rr_tr : Inport
  y_rr_tr : Inport  Port=2
  psi : Inport  Port=3
  Add : Sum
  Cos : Trigonometry  Operator=cos
  Cos1 : Trigonometry
  Product : Product
  Product1 : Product
  y_rr : Outport
  wires:
  Cos1/1 -> [sin_psi]
  Product/1 -> Add/1
  Cos/1 -> [cos_psi]
  Product1/1 -> Add/2
  psi/1 -> Cos1/1, Cos/1
  x_rr_tr/1 -> Product/2
  y_rr_tr/1 -> Product1/2
  Add/1 -> y_rr/1
  [cos_psi] -> Product1/1
  [sin_psi] -> Product/1

== matlab function main_model/Steering Assist Controller/Controller ==
  data: x0 input; u_ctrl output; U0 input; sv output; rmpcProps parameter; vehProps parameter; driverProps parameter; refTraj parameter
function [u_ctrl,sv] = fcn(x0, U0,rmpcProps,vehProps,driverProps,refTraj)
    u_ctrl=0;
    sv=0;
    coder.extrinsic('steerAssistController');
    [u_ctrl,sv]=steerAssistController(x0,U0,rmpcProps,vehProps,driverProps,refTraj);
end
